simulink model "sythese_sim"  (R2018b)
settings: Solver=VariableStepAuto  StartTime=0.0  StopTime=50  RelTol=1e-3
values from neighbouring files (symbols this model uses):
  alpha1 = 1    [synthese.m]
  alpha2 = 100    [synthese.m]
  r0 = x(3)    [aide_resolution_eq_bezout.m]
  r1 = x(4)    [aide_resolution_eq_bezout.m]
  r2 = x(5)    [aide_resolution_eq_bezout.m]
  sig0 = 1    [synthese.m]
  sig1 = 100    [synthese.m]
  sp1 = x(2)    [aide_resolution_eq_bezout.m]
  Te = 0.3    [aide_resolution_eq_bezout.m]    (also in synthese.m)
settings Model: Creator=poteaum  LastModifiedBy=poteaum

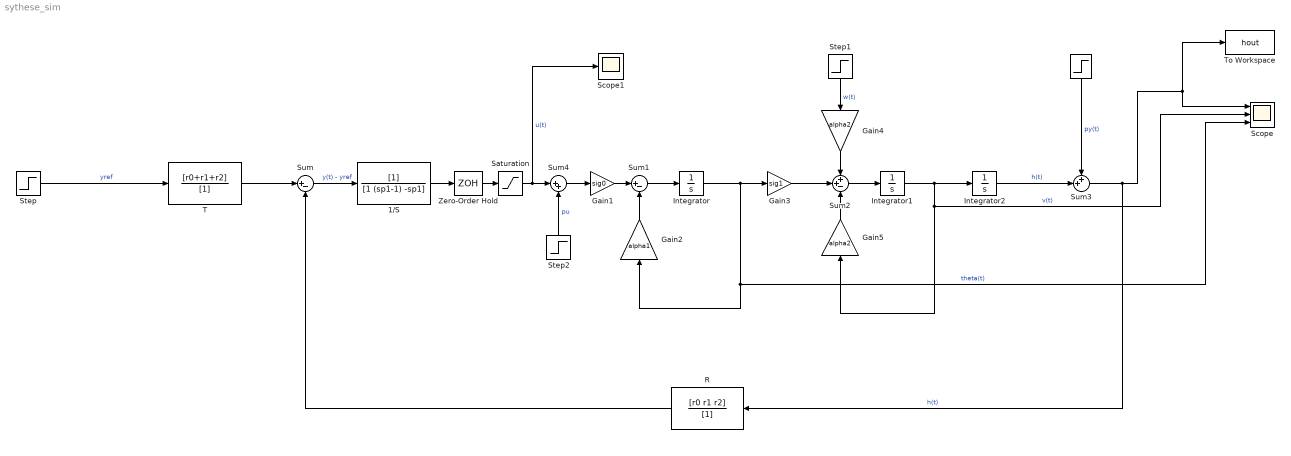
== system sythese_sim ==
  " " : Step  Time=0  After=0.1  SampleTime=0
  1/S : DiscreteFilter  Denominator=[1 (sp1-1) -sp1]
  Gain1 : Gain  Gain=sig0
  Gain2 : Gain  Gain=alpha1
  Gain3 : Gain  Gain=sig1
  Gain4 : Gain  Gain=alpha2
  Gain5 : Gain  Gain=alpha2
  Integrator : Integrator
  Integrator1 : Integrator
  Integrator2 : Integrator
  R : DiscreteFilter  Numerator=[r0 r1 r2]  Denominator=[1]
  Saturation : Saturate  UpperLimit=10  LowerLimit=-10
  Scope : Scope  NumInputPorts=3
  Scope1 : Scope
  Step : Step  Time=0  SampleTime=0
  Step1 : Step  Time=0  SampleTime=0
  Step2 : Step  Time=0  After=0.1  SampleTime=0
  Sum : Sum  Inputs=|+-
  Sum1 : Sum  Inputs=|+-
  Sum2 : Sum  Inputs=++-
  Sum3 : Sum  Inputs=++|
  Sum4 : Sum  Inputs=|++
  T : DiscreteFilter  Numerator=[r0+r1+r2]  Denominator=[1]  SampleTime=Te
  To Workspace : ToWorkspace  VariableName=hout  SaveFormat=Structure With Time  SampleTime=-1
  Zero-Order Hold : ZeroOrderHold  SampleTime=-1
  wires:
  Gain2/1 -> Sum1/2
  Sum1/1 -> Integrator/1
  Integrator/1 -> Gain2/1, Scope/3, Gain3/1  "theta(t)"
  Gain3/1 -> Sum2/2
  Gain4/1 -> Sum2/1
  Step1/1 -> Gain4/1  "w(t)"
  Sum2/1 -> Integrator1/1
  Gain5/1 -> Sum2/3
  Integrator1/1 -> Gain5/1, Scope/2, Integrator2/1  "v(t)"
  Integrator2/1 -> Sum3/2  "h(t)"
  Gain1/1 -> Sum1/1
  Sum/1 -> 1/S/1  "y(t) - yref"
  Step/1 -> T/1  "yref"
  Saturation/1 -> Sum4/1, Scope1/1  "u(t)"
  1/S/1 -> Zero-Order Hold/1
  Zero-Order Hold/1 -> Saturation/1
  R/1 -> Sum/2
  T/1 -> Sum/1
  Sum3/1 -> R/1, Scope/1, To Workspace/1  "h(t)"
  " "/1 -> Sum3/1  "py(t)"
  Sum4/1 -> Gain1/1
  Step2/1 -> Sum4/2  "pu"
